simulink subsystem "State_Machine_S2"  (R2023b)
settings: Solver=VariableStepAuto  StartTime=0.0  StopTime=10.0  RelTol=1e-3
settings Model: Creator=Inver  LastModifiedBy=Inver

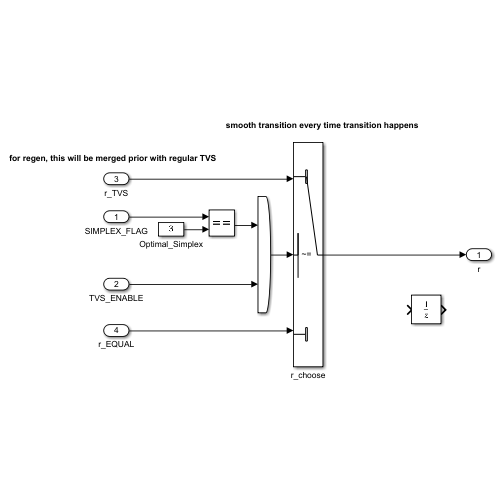
[thumbnail: Simulink's stored preview of the top-level diagram]
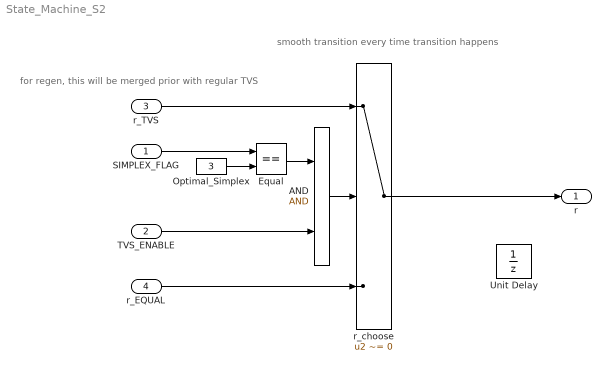
== system State_Machine_S2 ==
  note: for regen, this will be merged prior with regular TVS
  note: smooth transition every time transition happens
  SIMPLEX_FLAG : Inport
  TVS_ENABLE : Inport  Port=2
  r_TVS : Inport  Port=3
  r_EQUAL : Inport  Port=4
  AND : Logic  IconShape=distinctive  AllPortsSameDT=off  OutDataTypeStr=boolean
  Equal : RelationalOperator  Operator===  OutDataTypeStr=boolean  RndMeth=Simplest  InputSameDT=off
  Optimal_Simplex : Constant  Value=3
  Unit Delay : UnitDelay  SampleTime=-1  HasFrameUpgradeWarning=on
  r_choose : Switch  Criteria=u2 ~= 0  OutDataTypeStr=double  SaturateOnIntegerOverflow=off  InputSameDT=off
  r : Outport
  wires:
  TVS_ENABLE/1 -> AND/2
  Equal/1 -> AND/1
  r_choose/1 -> r/1
  SIMPLEX_FLAG/1 -> Equal/1
  Optimal_Simplex/1 -> Equal/2
  AND/1 -> r_choose/2
  r_TVS/1 -> r_choose/1
  r_EQUAL/1 -> r_choose/3
